simulink model "s0220a"  (Simulink 6.0)
settings: Solver=ode3  SolverMode=SingleTasking  StartTime=0.0  StopTime=900  FixedStep=1  MaxStep=1  RelTol=1e-3  AbsTol=1e-6
values from neighbouring files (symbols this model uses):
  Aabn = 1e-6*Aabn    (= 9e-06)    [m0220b.m]
  Aabv = 1e-6*Aabv    (= 6e-06)    [m0220b.m]
  Aspt = 500.    (= 500)    [m0220b.m]
  c1 = sqrt(2*g)/A    [m0208.m]    (also in m0218a.m = 5; m0218e.m = 10; m0220b.m; m0221a.m)
  c2 = cP/(rho*A)    (= 0.000666666666667)    [m0208.m]    (also in m0218a.m = 98.1; m0218e.m = 98.1; m0220b.m; m0221a.m)
settings Model: LastModifiedBy=Froriep
settings DataIOCC: LimitDataPoints=off  SaveOutput=off  TimeSaveName=t
settings OptimizationCC: BooleanDataType=off
settings DebuggingCC: SolverPrmCheckMsg=none
settings HardwareCC: TargetUnknown=on
settings GRTTargetCC: ModelReferenceCompliant=off  MatFileLogging=off

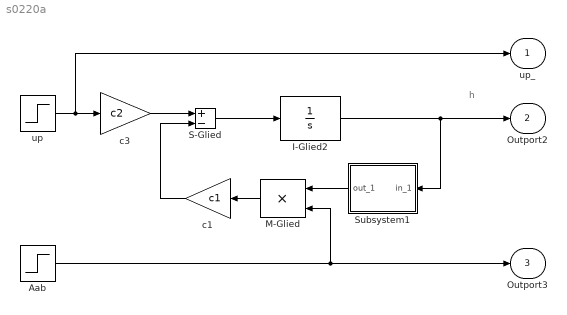
== system s0220a ==
  note: h
  Aab : Step  Time=Aspt  Before=Aabv  After=Aabn  SampleTime=0
  I-Glied2 : Integrator
  M-Glied : Product  Orientation=left  SaturateOnIntegerOverflow=on  RndMeth=Zero  InputSameDT=on
  S-Glied : Sum  Inputs=+-  SaturateOnIntegerOverflow=on  InputSameDT=on
  Subsystem1 : Subsystem  Orientation=left
      mask Display: disp('Wurzel')
  c1 : Gain  Orientation=left  Gain=c1  SaturateOnIntegerOverflow=on
  c3 : Gain  Gain=c2  SaturateOnIntegerOverflow=on
  up : Step  Time=50  After=4  SampleTime=0
  up_ : Outport
  Outport2 : Outport  Port=2
  Outport3 : Outport  Port=3
  wires:
  c3/1 -> S-Glied/1
  S-Glied/1 -> I-Glied2/1
  M-Glied/1 -> c1/1
  Subsystem1/1(out_1) -> M-Glied/1
  c1/1 -> S-Glied/2
  up/1 -> up_/1, c3/1
  I-Glied2/1 -> Outport2/1, Subsystem1/1(in_1)
  Aab/1 -> Outport3/1, M-Glied/2

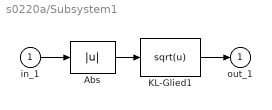
== system s0220a/Subsystem1 ==
  in_1 : Inport  Port=1  LatchInput=off
  Abs : Abs  SaturateOnIntegerOverflow=on
  KL-Glied1 : Fcn  Expr=sqrt(u)
  out_1 : Outport
  wires:
  KL-Glied1/1 -> out_1/1
  in_1/1 -> Abs/1
  Abs/1 -> KL-Glied1/1
